simulink model "model_153079011"  (Simulink 8.6)
settings: Solver=ode45  StartTime=0.0  StopTime=5  RelTol=1e-3
libraries: mblibv1 x12
settings Model: Creator=Ankit  LastModifiedBy=Akshay
settings DataIOCC: SignalLoggingSaveFormat=Dataset
settings OptimizationCC: ExpressionDepthLimit=128
settings DebuggingCC: UnderspecifiedInitializationDetection=Simplified  MergeDetectMultiDrivingBlocksExec=error  FcnCallInpInsideContextMsg=EnableAllAsError  StateNameClashWarn=none
settings GRTTargetCC: CombineOutputUpdateFcns=on  GRTInterface=off
settings ConfigComp: CovSFcnEnable=off
settings SimMechanicsCC: VisDuringSimulation=on
settings ConfigurationSet: Description=SimMechanics 2G

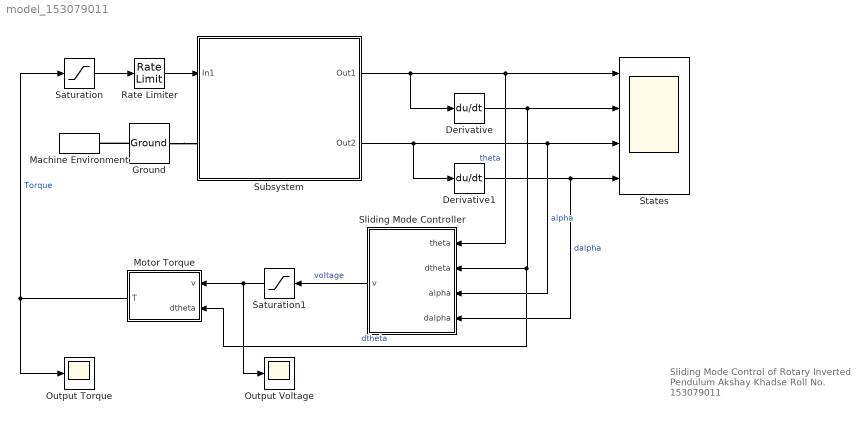
== system model_153079011 ==
  note: Sliding Mode Control of
      | Rotary Inverted Pendulum
      |
      | Akshay Khadse
      | Roll No. 153079011
  Derivative : Derivative
  Derivative1 : Derivative
  Ground : mblibv1/Bodies/Ground  UpdateFromCAD=off  LeftPortType=env  RightPortType=workingframe  PhysicalDomain=Mechanical  DialogClass=GroundBlock  CoordPosition=[0 0 0]  CoordPositionUnits=m  StateVectorMgrId=0  MachineId=[1 0]  ShowEnvPort=on  ParameterChecksum=[446715061, 509742564, 379883880, 889182031]  TopologyChecksum=[2724971321, 433967443, 3365040076, 3209492795]
  Machine Environment : mblibv1/Bodies/Machine Environment  Tag=Factory ground  PortType=env  PhysicalDomain=Mechanical  DialogTemplateClass=MECH.MachineEnvironment  SyncWhenCopied=off  Gravity=[0 0 -9.81]  GravityUnits=m/s^2  GravityAsSignal=off  Dimensionality=Auto-detect  AnalysisType=Forward dynamics  LinearAssemblyTolerance=1e-3  LinearAssemblyToleranceUnits=m  AngularAssemblyTolerance=1e-3  AngularAssemblyToleranceUnits=rad  ConstraintSolverType=Stabilizing  ConstraintRelTolerance=1e-4  ConstraintAbsTolerance=1e-4  UseRobustSingularityHandling=off  RedundancyAnalysisToleranceType=Automatically select tolerance  RedundancyAnalysisTolerance=1e-14  StatePerturbationType=Fixed  PerturbationSize=1e-5  VisualizeMachine=on  BodyVisualizationType=Use model default body geometries  BodyColorSelMode=Use model default  DefaultBodyColor=[1 0 0]
  Motor Torque : MATLAB Function  TreatAsAtomicUnit=on
  Output Torque : Scope
  Output Voltage : Scope
  Rate Limiter : RateLimiter
  Saturation : Saturate  UpperLimit=100  LowerLimit=-100  ZeroCross=off
  Saturation1 : Saturate  UpperLimit=10  LowerLimit=-10  ZeroCross=off
  Sliding Mode Controller : MATLAB Function  TreatAsAtomicUnit=on
  States : Scope  NumInputPorts=4
  Subsystem : Subsystem
      mask init:
      | throttle = imread('spe_mech_invpend.jpg');
      mask Display: image(throttle)
  wires:
  Rate Limiter/1 -> Subsystem/1(In1)
  Saturation/1 -> Rate Limiter/1
  Derivative/1 -> States/2, Motor Torque/2(dtheta), Sliding Mode Controller/2(dtheta)  "dtheta"
  Derivative1/1 -> Sliding Mode Controller/4(dalpha), States/4  "dalpha"
  Sliding Mode Controller/1(v) -> Saturation1/1  "voltage"
  Saturation1/1 -> Motor Torque/1(v), Output Voltage/1
  Motor Torque/1(T) -> Saturation/1, Output Torque/1  "Torque"
  Subsystem/2(Out2) -> Derivative1/1, Sliding Mode Controller/3(alpha), States/3  "alpha"
  Subsystem/1(Out1) -> Derivative/1, States/1, Sliding Mode Controller/1(theta)  "theta"
  connections:
  Ground/LConn1 -- Machine Environment/RConn1
  Ground/RConn1 -- Subsystem/LConn1

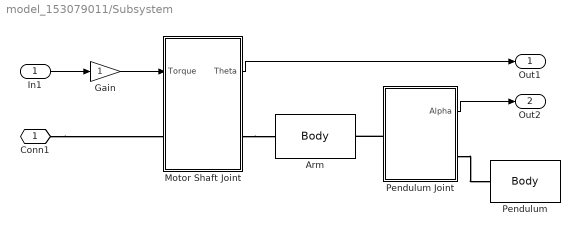
== system model_153079011/Subsystem ==
  In1 : Inport
  Arm : mblibv1/Bodies/Body  Tag=Factory generic  Description=Mechanical Blockset  LConnTagsString=CS1  RConnTagsString=CS2  UpdateFromCAD=off  DialogClass=MechanicalBodyBlock  Mass=0.028  MassUnits=kg  InertiaUnits=kg*m^2  Inertia=[0 0 0;0 0 0;0 0 0.000123]  Shape=Cylinder  ShapeDims=[1 1]  ShapeUnits=m  ShapeUse=false  Density=1  DensityUnits=kg/m^3  DensityUse=false  GraphicsMode=MACHINE_DEFAULT  BodyColorSelMode=MACHINE_DEFAULT  BodyColor=[1 0 0]  AttachedToCS=CG  CG=Left$CG$[0 0.08260/2 0]$CS1$CS1$m$[0 0 0]$Euler X-Y-Z$deg$WORLD$false$none  WorkingFrames=Left$CS1$[0 0 0]$WORLD$WORLD$m$[0 0 0]$Euler X-Y-Z$deg$WORLD$true$none#Right$CS2$[0 0.08260 0]$CS1$CS1$m$[0 0 0]$Euler X-Y-Z$deg$WORLD$true$none  CGPos=[0 0.08260/2 0]  CGRot=[0 0 0]  CS0Pos=[]  CS0Rot=[]  CS1Pos=[0 0 0]  CS1Rot=[0 0 0]  CS2Pos=[0 0.08260 0]  CS2Rot=[0 0 0]  CS3Pos=[]  CS3Rot=[]  CS4Pos=[]  CS4Rot=[]  CS5Pos=[]  CS5Rot=[]  CS6Pos=[]  CS6Rot=[]  CS7Pos=[]  CS7Rot=[]  CS8Pos=[]  CS8Rot=[]  CS9Pos=[]  CS9Rot=[]  CS10Pos=[]  CS10Rot=[]  CS11Pos=[]  CS11Rot=[]  CS12Pos=[]  CS12Rot=[]  CS13Pos=[]  CS13Rot=[]  CS14Pos=[]  CS14Rot=[]  CS15Pos=[]  CS15Rot=[]  CS16Pos=[]  CS16Rot=[]  CS17Pos=[]  CS17Rot=[]  CS18Pos=[]  CS18Rot=[]  CS19Pos=[]  CS19Rot=[]  CS20Pos=[]  CS20Rot=[]
  Gain : Gain
  Motor Shaft Joint : Subsystem
  Pendulum : mblibv1/Bodies/Body  Tag=Factory generic  Description=Mechanical Blockset  LConnTagsString=CS1  UpdateFromCAD=off  DialogClass=MechanicalBodyBlock  Mass=0.027  MassUnits=kg  InertiaUnits=kg*m^2  Inertia=[0 0 0;0 0 0;0 0 0.00011]  Shape=Cylinder  ShapeDims=[1 1]  ShapeUnits=m  ShapeUse=false  Density=1  DensityUnits=kg/m^3  DensityUse=false  GraphicsMode=MACHINE_DEFAULT  BodyColorSelMode=MACHINE_DEFAULT  BodyColor=[1 0 0]  AttachedToCS=CG  CG=Left$CG$[0 0 0.191/2]$CS1$CS1$m$[0 0 0]$Euler X-Y-Z$deg$WORLD$false$none  WorkingFrames=Left$CS1$[0 0 0]$ADJOINING$ADJOINING$m$[0 0 0]$Euler X-Y-Z$deg$WORLD$true$none#Right$CS2$[0 0 0.191]$CS1$CS1$m$[0 0 0]$Euler X-Y-Z$deg$WORLD$false$none  CGPos=[0 0 0.191/2]  CGRot=[0 0 0]  CS0Pos=[]  CS0Rot=[]  CS1Pos=[0 0 0]  CS1Rot=[0 0 0]  CS2Pos=[0 0 0.191]  CS2Rot=[0 0 0]  CS3Pos=[]  CS3Rot=[]  CS4Pos=[]  CS4Rot=[]  CS5Pos=[]  CS5Rot=[]  CS6Pos=[]  CS6Rot=[]  CS7Pos=[]  CS7Rot=[]  CS8Pos=[]  CS8Rot=[]  CS9Pos=[]  CS9Rot=[]  CS10Pos=[]  CS10Rot=[]  CS11Pos=[]  CS11Rot=[]  CS12Pos=[]  CS12Rot=[]  CS13Pos=[]  CS13Rot=[]  CS14Pos=[]  CS14Rot=[]  CS15Pos=[]  CS15Rot=[]  CS16Pos=[]  CS16Rot=[]  CS17Pos=[]  CS17Rot=[]  CS18Pos=[]  CS18Rot=[]  CS19Pos=[]  CS19Rot=[]  CS20Pos=[]  CS20Rot=[]
  Pendulum Joint : Subsystem
  Conn1 : PMIOPort  Port=1  Side=Left
  Out1 : Outport
  Out2 : Outport  Port=2
  wires:
  Motor Shaft Joint/1(Theta) -> Out1/1
  In1/1 -> Gain/1
  Pendulum Joint/1(Alpha) -> Out2/1
  Gain/1 -> Motor Shaft Joint/1(Torque)
  connections:
  Motor Shaft Joint/RConn1 -- Arm/LConn1
  Pendulum Joint/LConn1 -- Arm/RConn1
  Pendulum Joint/RConn1 -- Pendulum/LConn1
  Conn1/RConn1 -- Motor Shaft Joint/LConn1

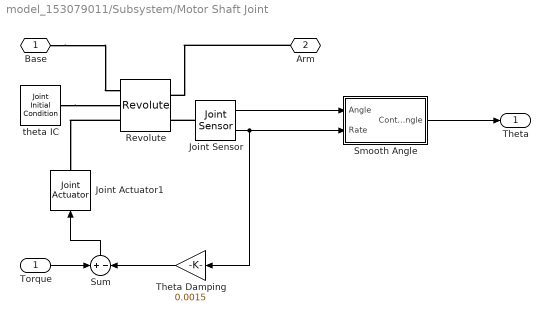
== system model_153079011/Subsystem/Motor Shaft Joint ==
  Torque : Inport
  Joint Actuator1 : mblibv1/Sensors &  Actuators/Joint Actuator  UpdateFromCAD=off  PhysicalDomain=Mechanical  PortType=blob  ActuationStyle=Force  AngleUnits=deg  ArcVelocityUnits=deg/s  ArcAccelerationUnits=deg/s^2  CoordPositionUnits=m  VelocityUnits=m/s  AccelerationUnits=m/s^2  ForceUnits=N  TorqueUnits=N-m  ActiveIO=on  Width=1  DialogClass=MechanicalActuatorBlock  Primitive=R1  ReferenceFrame=Absolute (World)
  Joint Sensor : mblibv1/Sensors &  Actuators/Joint Sensor  Description=Mechanical Blockset  UpdateFromCAD=off  PhysicalDomain=Mechanical  PortType=blob  Muxed=off  Pose=off  Angle=on  AngleUnits=deg  ArcVelocity=on  ArcVelocityUnits=rad/s  ArcAcceleration=off  ArcAccelerationUnits=deg/s^2  CoordPosition=on  CoordPositionUnits=m  Velocity=off  VelocityUnits=m/s  Acceleration=off  AccelerationUnits=m/s^2  Quaternion=on  QuaternionDT=off  QuaternionDDT=off  QuaternionUnits=off  OutputVector=[ 1 1 ]  ActiveIO=on  Width=2  DialogClass=MechanicalSensorBlock  Primitive=R1  Force=off  ForceUnits=N  Torque=off  TorqueUnits=N*m  ReferenceFrame=Absolute (INERTIAL)  ReactionSensedSide=Base  ReactionReferenceFrame=Absolute (World)  ReactionForce=off  ReactionForceUnits=N  ReactionMoment=off  ReactionMomentUnits=N*m
  Revolute : mblibv1/Joints/Revolute  Tag=Factory generic  Description=Mechanical Blockset  LConnTagsString=__newl0|SA1|SA2  RConnTagsString=__newr0|SA1  UpdateFromCAD=off  NumSAPorts=3  CutJoint=off  MarkAsCut=off  Primitives=revolute  PrimitiveProps=R1$Base$[0 0 1]$revolute  DialogClass=JointBlock  R1Axis=[0 0 1]
  Smooth Angle : Subsystem  mask{rad=deg, rads=rad/s}
      mask prompts: rad "Angle measured in:"; rads "Rate measured in:"
      mask help: Constructs continuous angle from angular velocity rate and piecewise continuous angle measured by Joint Sensor on a revolute primitive. Integrates angular velocity to determine number of revolutions that the joint primitive has undergone.
      mask TypeOptions rad: rad | deg
      mask TypeOptions rads: rad/s | deg/s
  Sum : Sum  Inputs=+|-  SaturateOnIntegerOverflow=on  InputSameDT=on  OutDataTypeStr=Inherit: Same as first input
  Theta Damping : Gain  Gain=0.0015  SaturateOnIntegerOverflow=on  OutDataTypeStr=Inherit: Same as input  ParamDataTypeStr=Inherit: Same as input
  theta IC : mblibv1/Sensors &  Actuators/Joint Initial Condition  Description=Mechanical Blockset  UpdateFromCAD=off  LeftPortType=blob  RightPortType=blob  PhysicalDomain=Mechanical  DialogClass=InitialConditionBlock  Primitive=R1  CoordPosition=0  Velocity=0.0  AngleUnits=deg  ArcVelocityUnits=deg/s  CoordPositionUnits=m  VelocityUnits=m/s  InitialConditions=P1$false$0$m$rad$0$m/s$rad/s#P2$false$0$m$rad$0$m/s$rad/s#P3$false$0$m$rad$0$m/s$rad/s#R1$true$0$m$deg$0.0$m/s$deg/s#R2$false$0$m$rad$0$m/s$rad/s#R3$false$0$m$rad$0$m/s$rad/s#S$false$0$m$rad$0$m/s$rad/s  P1PIC=0  P1VIC=0  P2PIC=0  P2VIC=0  P3PIC=0  P3VIC=0  R1PIC=0  R1VIC=0.0  R2PIC=0  R2VIC=0  R3PIC=0  R3VIC=0  SPIC=0  SVIC=0
  Base : PMIOPort  Port=1  Side=Left
  Arm : PMIOPort  Port=2  Side=Right
  Theta : Outport
  wires:
  Joint Sensor/2 -> Smooth Angle/2(Rate), Theta Damping/1
  Torque/1 -> Sum/1
  Theta Damping/1 -> Sum/2
  Sum/1 -> Joint Actuator1/1
  Joint Sensor/1 -> Smooth Angle/1(Angle)
  Smooth Angle/1(Continuous Angle) -> Theta/1
  connections:
  Joint Sensor/LConn1 -- Revolute/RConn2
  Revolute/LConn3 -- Joint Actuator1/RConn1
  theta IC/RConn1 -- Revolute/LConn2
  Arm/RConn1 -- Revolute/RConn1
  Base/RConn1 -- Revolute/LConn1

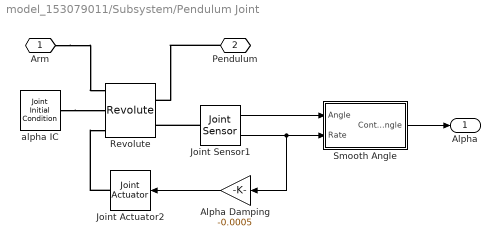
== system model_153079011/Subsystem/Pendulum Joint ==
  Alpha Damping : Gain  Gain=-0.0005  SaturateOnIntegerOverflow=on  OutDataTypeStr=Inherit: Same as input  ParamDataTypeStr=Inherit: Same as input
  Joint Actuator2 : mblibv1/Sensors &  Actuators/Joint Actuator  Description=Mechanical Blockset  UpdateFromCAD=off  PhysicalDomain=Mechanical  PortType=blob  ActuationStyle=Force  AngleUnits=deg  ArcVelocityUnits=deg/s  ArcAccelerationUnits=deg/s^2  CoordPositionUnits=m  VelocityUnits=m/s  AccelerationUnits=m/s^2  ForceUnits=N  TorqueUnits=N-m  ActiveIO=on  Width=1  DialogClass=MechanicalActuatorBlock  Primitive=R1  ReferenceFrame=Absolute (INERTIAL)
  Joint Sensor1 : mblibv1/Sensors &  Actuators/Joint Sensor  Description=Mechanical Blockset  UpdateFromCAD=off  PhysicalDomain=Mechanical  PortType=blob  Muxed=off  Pose=off  Angle=on  AngleUnits=deg  ArcVelocity=on  ArcVelocityUnits=rad/s  ArcAcceleration=off  ArcAccelerationUnits=deg/s^2  CoordPosition=on  CoordPositionUnits=m  Velocity=off  VelocityUnits=m/s  Acceleration=off  AccelerationUnits=m/s^2  Quaternion=on  QuaternionDT=off  QuaternionDDT=off  QuaternionUnits=off  OutputVector=[ 1 1 ]  ActiveIO=on  Width=2  DialogClass=MechanicalSensorBlock  Primitive=R1  Force=off  ForceUnits=N  Torque=off  TorqueUnits=N*m  ReferenceFrame=Absolute (INERTIAL)  ReactionSensedSide=Base  ReactionReferenceFrame=Absolute (World)  ReactionForce=off  ReactionForceUnits=N  ReactionMoment=off  ReactionMomentUnits=N*m
  Revolute : mblibv1/Joints/Revolute  Tag=Factory generic  Description=Mechanical Blockset  LConnTagsString=__newl0|SA1|SA2  RConnTagsString=__newr0|SA1  UpdateFromCAD=off  NumSAPorts=3  CutJoint=off  MarkAsCut=off  Primitives=revolute  PrimitiveProps=R1$Base$[0 1 0]$revolute  DialogClass=JointBlock  R1Axis=[0 1 0]
  Smooth Angle : Subsystem  mask{rad=deg, rads=rad/s}
      mask prompts: rad "Angle measured in:"; rads "Rate measured in:"
      mask help: Constructs continuous angle from angular velocity rate and piecewise continuous angle measured by Joint Sensor on a revolute primitive. Integrates angular velocity to determine number of revolutions that the joint primitive has undergone.
      mask TypeOptions rad: rad | deg
      mask TypeOptions rads: rad/s | deg/s
  alpha IC : mblibv1/Sensors &  Actuators/Joint Initial Condition  Description=Mechanical Blockset  UpdateFromCAD=off  LeftPortType=blob  RightPortType=blob  PhysicalDomain=Mechanical  DialogClass=InitialConditionBlock  Primitive=R1  CoordPosition=25  Velocity=0.0  AngleUnits=deg  ArcVelocityUnits=deg/s  CoordPositionUnits=m  VelocityUnits=m/s  InitialConditions=P1$false$0$m$rad$0$m/s$rad/s#P2$false$0$m$rad$0$m/s$rad/s#P3$false$0$m$rad$0$m/s$rad/s#R1$true$25$m$deg$0.0$m/s$deg/s#R2$false$0$m$rad$0$m/s$rad/s#R3$false$0$m$rad$0$m/s$rad/s#S$false$0$m$rad$0$m/s$rad/s  P1PIC=0  P1VIC=0  P2PIC=0  P2VIC=0  P3PIC=0  P3VIC=0  R1PIC=25  R1VIC=0.0  R2PIC=0  R2VIC=0  R3PIC=0  R3VIC=0  SPIC=0  SVIC=0
  Arm : PMIOPort  Port=1  Side=Left
  Pendulum : PMIOPort  Port=2  Side=Right
  Alpha : Outport
  wires:
  Joint Sensor1/1 -> Smooth Angle/1(Angle)
  Joint Sensor1/2 -> Smooth Angle/2(Rate), Alpha Damping/1
  Smooth Angle/1(Continuous Angle) -> Alpha/1
  Alpha Damping/1 -> Joint Actuator2/1
  connections:
  Joint Sensor1/LConn1 -- Revolute/RConn2
  alpha IC/RConn1 -- Revolute/LConn2
  Joint Actuator2/RConn1 -- Revolute/LConn3
  Arm/RConn1 -- Revolute/LConn1
  Pendulum/RConn1 -- Revolute/RConn1

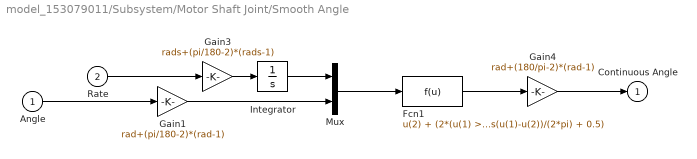
== system model_153079011/Subsystem/Motor Shaft Joint/Smooth Angle ==
  Angle : Inport
  Rate : Inport  Port=2
  Fcn1 : Fcn  Expr=u(2) + (2*(u(1) > u(2)) - 1)*2*pi*floor(abs(u(1)-u(2))/(2*pi) + 0.5)
  Gain1 : Gain  Gain=rad+(pi/180-2)*(rad-1)  SaturateOnIntegerOverflow=on  OutDataTypeStr=Inherit: Same as input  ParamDataTypeStr=Inherit: Same as input
  Gain3 : Gain  Gain=rads+(pi/180-2)*(rads-1)  SaturateOnIntegerOverflow=on  OutDataTypeStr=Inherit: Same as input  ParamDataTypeStr=Inherit: Same as input
  Gain4 : Gain  Gain=rad+(180/pi-2)*(rad-1)  SaturateOnIntegerOverflow=on  OutDataTypeStr=Inherit: Same as input  ParamDataTypeStr=Inherit: Same as input
  Integrator : Integrator  AbsoluteTolerance=1e-3
  Mux : Mux  Inputs=2
  Continuous Angle : Outport
  wires:
  Gain1/1 -> Mux/2
  Gain3/1 -> Integrator/1
  Integrator/1 -> Mux/1
  Mux/1 -> Fcn1/1
  Fcn1/1 -> Gain4/1
  Rate/1 -> Gain3/1
  Angle/1 -> Gain1/1
  Gain4/1 -> Continuous Angle/1

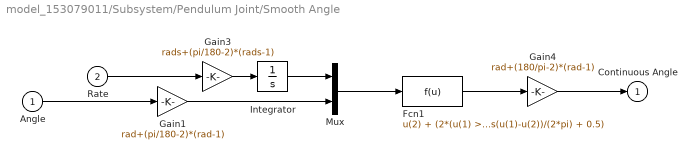
== system model_153079011/Subsystem/Pendulum Joint/Smooth Angle ==
  Angle : Inport
  Rate : Inport  Port=2
  Fcn1 : Fcn  Expr=u(2) + (2*(u(1) > u(2)) - 1)*2*pi*floor(abs(u(1)-u(2))/(2*pi) + 0.5)
  Gain1 : Gain  Gain=rad+(pi/180-2)*(rad-1)  SaturateOnIntegerOverflow=on  OutDataTypeStr=Inherit: Same as input  ParamDataTypeStr=Inherit: Same as input
  Gain3 : Gain  Gain=rads+(pi/180-2)*(rads-1)  SaturateOnIntegerOverflow=on  OutDataTypeStr=Inherit: Same as input  ParamDataTypeStr=Inherit: Same as input
  Gain4 : Gain  Gain=rad+(180/pi-2)*(rad-1)  SaturateOnIntegerOverflow=on  OutDataTypeStr=Inherit: Same as input  ParamDataTypeStr=Inherit: Same as input
  Integrator : Integrator  AbsoluteTolerance=1e-3
  Mux : Mux  Inputs=2
  Continuous Angle : Outport
  wires:
  Gain1/1 -> Mux/2
  Gain3/1 -> Integrator/1
  Integrator/1 -> Mux/1
  Mux/1 -> Fcn1/1
  Fcn1/1 -> Gain4/1
  Rate/1 -> Gain3/1
  Angle/1 -> Gain1/1
  Gain4/1 -> Continuous Angle/1

== matlab function Motor Torque ==
  data: v input double; T output double; dtheta input double
function T = fcn(v, dtheta)
%% Convert angles to radians
dtheta=dtheta*(pi/180);

%% Motor Parameters
kt=0.1119;
km=0.02797;
rm=3.3;

%% Output Torque
T = kt*(v-km*dtheta)/rm;

== matlab function Sliding Mode Controller ==
  data: theta input double; v output double; dtheta input double; alpha input double; dalpha input double
function v = fcn(theta,dtheta,alpha,dalpha)

%% Convert Angles to radians
theta=theta*(pi/180);
dtheta=dtheta*(pi/180);
alpha=alpha*(pi/180);
dalpha=dalpha*(pi/180);

%% Model Parameters
kt=0.02797;
km=0.02797;
rm=3.3;
L=0.153;
r=0.08260;
jeq=1.23*10^-4+0.00011;
m=0.027;
beq=0.0015;

%% Tuning Parameters
k=2;
lambda1=0.2;
lambda2=0.01;
lambda3=5;
phi=0.5;

%k=3;
%lambda1=0.5;
%lambda2=0.01;
%lambda3=10;
%phi=0.3;

%% Model
a=jeq+m*r*r;
b=m*L*r;
c=4*m*L*L/3;
d=m*9.81*L;
g=(kt*km+beq*rm)/rm;


f1=(-(b^2/2)*sin(2*alpha)*dalpha^2 - g*b*dtheta*cos(alpha) + a*d*sin(alpha))/(a*c-b^2*(cos(alpha))^2);
g1=kt*b*cos(alpha)/(rm*(a*c-b^2*(cos(alpha))^2));
f2=(c*f1-d*sin(alpha))/(b*cos(alpha));
g2=kt*c/(rm*(a*c-b^2*(cos(alpha))^2));

%% Manifolds and Lyapunov Function
s1 = dalpha + lambda1*alpha;
s2 = dtheta + lambda3*theta;
v = abs(s1) + lambda2*abs(s2);

%% Saturation
if(phi<abs(v))
    out=v/phi;
else
    out=sign(v);
end

%% Output Voltage
v = (-k*out-(lambda1*dalpha+f1)*sign(s1)-lambda2*(lambda3*dtheta+f2)*sign(s2))/(g1*sign(s1)+lambda2*g2*sign(s2));
